simulink model "Gain_model_wI"  (R2023b)
settings: Solver=FixedStepAuto  StartTime=0.0  StopTime=30  FixedStep=1  RelTol=1e-3
settings Model: PacingRate=1.050000  Creator=20181234  LastModifiedBy=20181234
settings OptimizationCC: ReuseModelBlockBuffer=off

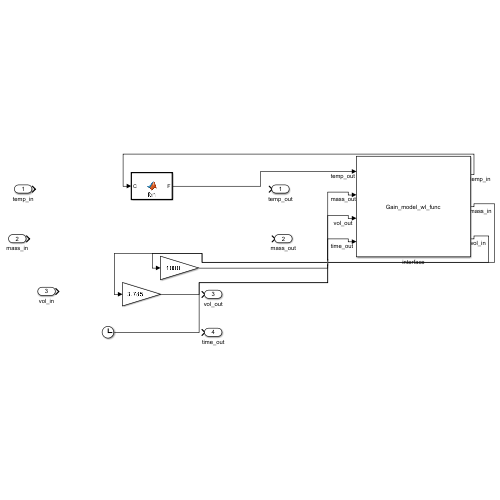
[thumbnail: Simulink's stored preview of the top-level diagram]
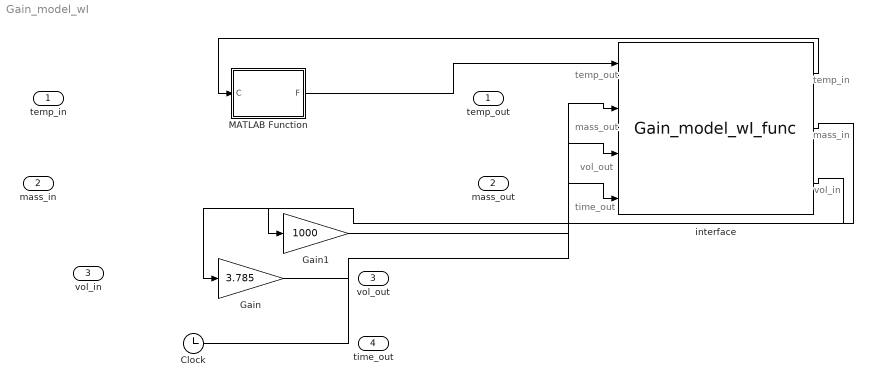
== system Gain_model_wI ==
  note: temp_out
  note: mass_out
  note: vol_out
  note: time_out
  note: temp_in
  note: mass_in
  note: vol_in
  temp_in : Inport
  mass_in : Inport  Port=2
  vol_in : Inport  Port=3
  Clock : Clock
  Gain : Gain  Gain=3.785
  Gain1 : Gain  Gain=1000
  MATLAB Function : MATLAB Function  TreatAsAtomicUnit=on
  interface : M-S-Function  FunctionName=Gain_model_wI_func
  temp_out : Outport
  mass_out : Outport  Port=2
  vol_out : Outport  Port=3
  time_out : Outport  Port=4
  wires:
  interface/1 -> MATLAB Function/1(C)
  MATLAB Function/1(F) -> interface/1
  Gain1/1 -> interface/2
  interface/2 -> Gain1/1
  interface/3 -> Gain/1
  Gain/1 -> interface/3
  Clock/1 -> interface/4

== matlab function Gain_model_wI/MATLAB Function ==
  data: C input; F output
function F = fcn(C)

F = (C*9/5)+32;
